simulink model "Q_method"  (R2024b)
settings: Solver=VariableStepAuto  StartTime=0.0  StopTime=10.0  RelTol=1e-3
settings Model: Creator=esteb  LastModifiedBy=esteb

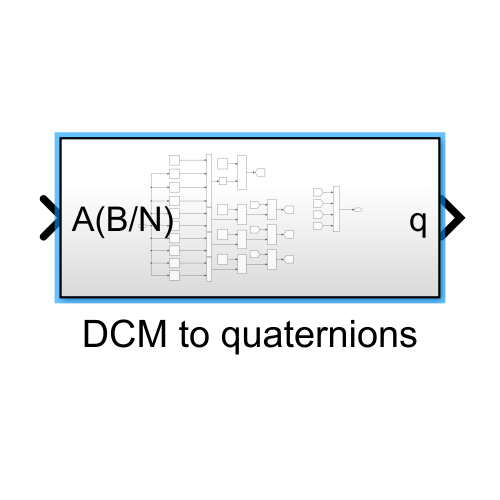
[thumbnail: Simulink's stored preview of the top-level diagram]
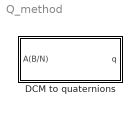
== system Q_method ==
  DCM to quaternions : Subsystem

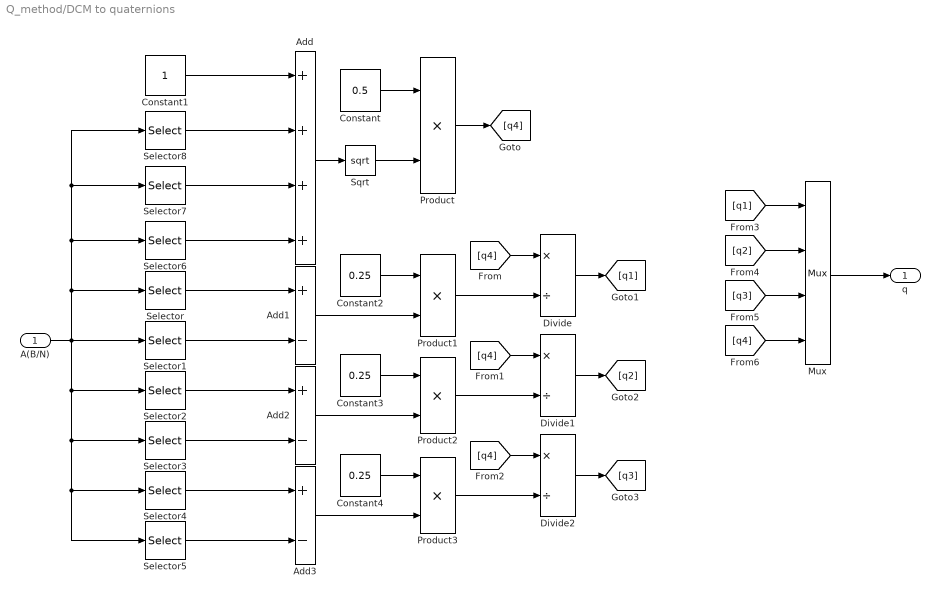
== system Q_method/DCM to quaternions ==
  A(B/N) : Inport
  Add : Sum  Inputs=++++
  Add1 : Sum  Inputs=+-
  Add2 : Sum  Inputs=+-
  Add3 : Sum  Inputs=+-
  Constant : Constant  Value=0.5
  Constant1 : Constant
  Constant2 : Constant  Value=0.25
  Constant3 : Constant  Value=0.25
  Constant4 : Constant  Value=0.25
  Divide : Product  Inputs=*/
  Divide1 : Product  Inputs=*/
  Divide2 : Product  Inputs=*/
  Mux : Mux
  Product{,1..3} (4 alike) : Product
  Selector : Selector  NumberOfDimensions=2  InputPortWidth=3  IndexOptions=Index vector (dialog),Index vector (dialog)  Indices=2,3  OutputSizes=1,1
  Selector1 : Selector  NumberOfDimensions=2  InputPortWidth=3  IndexOptions=Index vector (dialog),Index vector (dialog)  Indices=3,2  OutputSizes=1,1
  Selector2 : Selector  NumberOfDimensions=2  InputPortWidth=3  IndexOptions=Index vector (dialog),Index vector (dialog)  Indices=3,1  OutputSizes=1,1
  Selector3 : Selector  NumberOfDimensions=2  InputPortWidth=3  IndexOptions=Index vector (dialog),Index vector (dialog)  Indices=1,3  OutputSizes=1,1
  Selector4 : Selector  NumberOfDimensions=2  InputPortWidth=3  IndexOptions=Index vector (dialog),Index vector (dialog)  Indices=1,2  OutputSizes=1,1
  Selector5 : Selector  NumberOfDimensions=2  InputPortWidth=3  IndexOptions=Index vector (dialog),Index vector (dialog)  Indices=2,1  OutputSizes=1,1
  Selector6 : Selector  NumberOfDimensions=2  InputPortWidth=3  IndexOptions=Index vector (dialog),Index vector (dialog)  Indices=3,3  OutputSizes=1,1
  Selector7 : Selector  NumberOfDimensions=2  InputPortWidth=3  IndexOptions=Index vector (dialog),Index vector (dialog)  Indices=2,2  OutputSizes=1,1
  Selector8 : Selector  NumberOfDimensions=2  InputPortWidth=3  IndexOptions=Index vector (dialog),Index vector (dialog)  Indices=1,1  OutputSizes=1,1
  Sqrt : Sqrt
  q : Outport
  wires:
  Mux/1 -> q/1
  Product2/1 -> Divide1/2
  Divide2/1 -> [q3]
  Add1/1 -> Product1/2
  [q3] -> Mux/3
  [q4] -> Mux/4
  [q1] -> Mux/1
  Add3/1 -> Product3/2
  [q4] -> Divide1/1
  Constant2/1 -> Product1/1
  Selector/1 -> Add1/1
  Product1/1 -> Divide/2
  Constant/1 -> Product/1
  Selector8/1 -> Add/2
  Selector2/1 -> Add2/1
  Add/1 -> Sqrt/1
  Divide/1 -> [q1]
  Selector4/1 -> Add3/1
  Selector3/1 -> Add2/2
  Constant4/1 -> Product3/1
  [q2] -> Mux/2
  A(B/N)/1 -> Selector4/1, Selector5/1, Selector3/1, Selector2/1, Selector/1, Selector6/1, Selector7/1, Selector8/1, Selector1/1
  Sqrt/1 -> Product/2
  Selector5/1 -> Add3/2
  [q4] -> Divide/1
  [q4] -> Divide2/1
  Add2/1 -> Product2/2
  Selector6/1 -> Add/4
  Selector7/1 -> Add/3
  Selector1/1 -> Add1/2
  Constant3/1 -> Product2/1
  Constant1/1 -> Add/1
  Divide1/1 -> [q2]
  Product/1 -> [q4]
  Product3/1 -> Divide2/2
